simulink model "ADSBMonitor"  (R2022a)
settings: Solver=FixedStepDiscrete  StartTime=0.0  StopTime=10  RelTol=1e-3
PreLoadFcn:
  | radioSampleRate = 2.4e6;
  | adsbParam = helperAdsbConfig(radioSampleRate);
  | load dataAdsbBusObjects
  | LaunchMap = 0;
  | LogData = 0;
  | BaudRate=9600;
InitFcn:
  | load dataAdsbBusObjects
  | helperAdsbCheckModelParams;
libraries: simulink x2, ADSBExampleLib x2, commsource2 x1, sdrrlib x1
CloseFcn:
  | hFig = findall(0, 'Type', 'figure', 'Tag', 'ADS-B Aircraft Tracking');
  | if ishghandle(hFig)
  | close(hFig);
  | end
  | clear hFig
settings Model: Creator=The MathWorks, Inc.  LastModifiedBy=Michael
settings SolverCC: AlgebraicLoopSolver=TrustRegion
settings DataIOCC: LimitDataPoints=on  SaveFormat=Array  SaveOutput=off  SaveTime=off  ReturnWorkspaceOutputs=off
settings OptimizationCC: BooleanDataType=off  DefaultParameterBehavior=Inlined  LocalBlockOutputs=off  LifeSpan=inf
settings DebuggingCC: AlgebraicLoopMsg=error  SingleTaskRateTransMsg=error  UnconnectedInputMsg=warning  UnconnectedOutputMsg=warning  UnconnectedLineMsg=warning  AllowSymbolicDim=off  SFUnexpectedBacktrackingDiag=warning  SFNoUnconditionalDefaultTransitionDiag=warning  SFExecutionAtInitializationDiag=none  SFMachineParentedDataDiag=warning  ArithmeticOperatorsInVariantConditions=warning
settings ModelReferenceCC: PropagateSignalLabelsOutOfModel=off
settings SFSimCC: SimUseLocalCustomCode=off  CustomCodeUndefinedFunction=UseInterfaceOnly
settings RTWCC: RTWUseLocalCustomCode=off  DLArmComputeVersion=19.05
settings CodeAppCC: StateflowObjectComments=on
settings GRTTargetCC: TargetLangStandard=C89/C90 (ANSI)
settings ConfigComp: CovScope=ReferencedModels  CovMetricSettings=dw  CovSaveCumulativeToWorkspaceVar=on  CovSaveSingleToWorkspaceVar=on  CovExternalEMLEnable=off  CovSFcnEnable=off

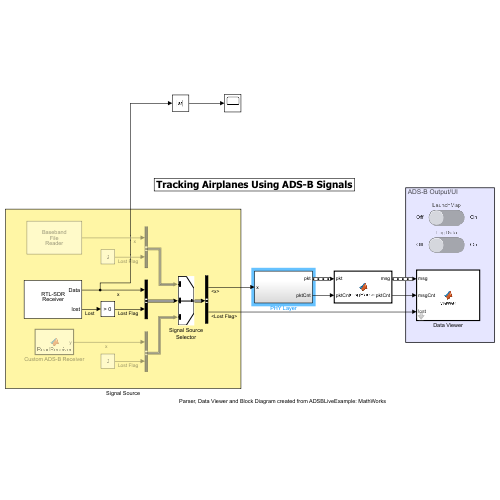
[thumbnail: Simulink's stored preview of the top-level diagram]
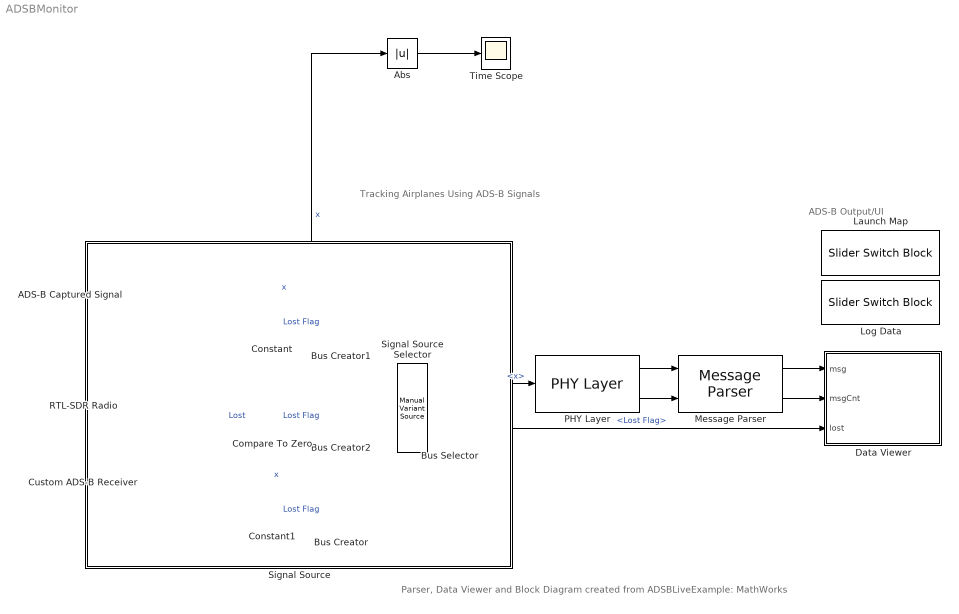
== system ADSBMonitor ==
  note: ADS-B Output/UI
  note: Tracking Airplanes Using ADS-B Signals
  note: Parser, Data Viewer and Block Diagram created from ADSBLiveExample: MathWorks
  ADS-B Captured Signal : commsource2/Baseband File Reader  Filename=adsb_capture_01.bb  InheritSampleTimeFromFile=on  SampleTime=1  SamplesPerFrame=adsbParam.SamplesPerFrame  CyclicRepetition=on  FileEndOutputPort=off  SimulateUsing=Code generation
      settings: SourceProductBaseCode=CM
  Abs : Abs  SaturateOnIntegerOverflow=off
  Bus Creator : BusCreator  Inputs=2
  Bus Creator1 : BusCreator  Inputs=2
  Bus Creator2 : BusCreator  Inputs=2
  Bus Selector : BusSelector  OutputSignals=x,Lost Flag
  Compare To Zero : simulink/Logic and Bit Operations/Compare To Zero  relop=>  OutDataTypeStr=boolean
  Constant : Constant  Value=0
  Constant1 : Constant  Value=0
  Custom ADS-B Receiver : MATLAB Function  TreatAsAtomicUnit=on
  Data Viewer : MATLAB Function  StopFcn=|  TreatAsAtomicUnit=on  mask(ADS-B viewer){logfilename=test.txt}
      | adsbGUI=findall(0,'type','figure','Tag','ADS-B Aircraft Tracking');
      | if ~isempty(adsbGUI)
      |   viewer=getappdata(adsbGUI,'ViewerHandle');
      |   stop(viewer);
      | end
      mask prompts: logfilename "Log data to file :"
  Launch Map : SliderSwitchBlock
      settings: Values={{'Off', 'On'}, [0 1]}
  Log Data : SliderSwitchBlock
      settings: Values={{'Off', 'On'}, [0 1]}
  Message Parser : ADSBExampleLib/Message Parser  SystemSampleTime=-1  VariantActivationTime=update diagram  Latency=0  AutoFrameSizeCalculation=off
  PHY Layer : ADSBExampleLib/PHY Layer  SystemSampleTime=-1  VariantActivationTime=update diagram  Latency=0  AutoFrameSizeCalculation=off
  RTL-SDR Radio : sdrrlib/RTL-SDR Receiver  IPAddress=0  CenterFrequencySource=Dialog  CenterFrequency=1090e6  GainSource=Dialog  Gain=60  ADCRate=adsbParam.FrontEndSampleRate  FrequencyCorrection=0  LostSamplesOutputPort=on  LatencyOutputPort=off  OutputDataType=single  FrameLength=adsbParam.SamplesPerFrame  EnableBurstMode=off  NumFramesInBurst=100  sobjType=sdrr.internal.SDRRTLReceiverSL  dataUDPPort=-1  ctrlUDPPort=-1  subDeviceList=nosubdev  sdrBlockType=SDRBlockTypeSLT.SDRRxBlock  requester=UNUSED_BY_SFCN  sdrExecutionMode=SDRExecutionModeSLT.ExecModeHW  BypassUserLogic=off  DecimatorSelect=DDC decimator  SourceSelect=RF data  SineAmplitude=16000  EnableInternalClock=off  BypassIQBalance=off  IFBandwidth=40e6  ADCRateSource=Dialog  IntermediateFrequency=0  DecimationFactorSource=Dialog  DecimationFactor=512  RFFrequencyIsTunable=logical(0)  SampleTime=(adsbParam.SamplesPerFrame)/(adsbParam.FrontEndSampleRate)  IFBandwidthSource=Dialog  SineFrequency=30000  BypassDCBlockingFilter=off  IntermediateFrequencySource=Dialog  IQBalanceCoefficients=64  SkipAllHardwareResetAndInitialization=off  EnableIQCalibrationTable=on  CacheIQCalibrationTable=off  EnableOffsetTuning=off  EnableRTLAGC=off  EnableTestMode=off  EnableTunerAGC=off  FrequencyCorrectionSource=Dialog  NumMLBuffers=128  NumUSBBuffers=16  RTLCrystalFrequency=28800000  TunerCrystalFrequency=28800000
      settings: SourceProductBaseCode=RTLSDR
  Signal Source : Subsystem
      mask Display: disp('')
  Signal Source Selector : simulink/Signal Routing/Manual Variant Source  NumChoices=3  LabelModeActiveChoice=V_2
  Time Scope : Scope
  wires:
  Message Parser/1 -> Data Viewer/1(msg)
  Message Parser/2 -> Data Viewer/2(msgCnt)
  PHY Layer/1 -> Message Parser/1
  PHY Layer/2 -> Message Parser/2
  Bus Selector/2 -> Data Viewer/3(lost)  "<Lost Flag>"
  Bus Selector/1 -> PHY Layer/1  "<x>"
  RTL-SDR Radio/1 -> Abs/1, Bus Creator2/1  "x"
  ADS-B Captured Signal/1 -> Bus Creator1/1  "x"
  Bus Creator2/1 -> Signal Source Selector/2
  Custom ADS-B Receiver/1(y) -> Bus Creator/1  "x"
  Signal Source Selector/1 -> Bus Selector/1
  Bus Creator/1 -> Signal Source Selector/3
  Bus Creator1/1 -> Signal Source Selector/1
  RTL-SDR Radio/2 -> Compare To Zero/1  "Lost"
  Compare To Zero/1 -> Bus Creator2/2  "Lost Flag"
  Constant/1 -> Bus Creator1/2  "Lost Flag"
  Constant1/1 -> Bus Creator/2  "Lost Flag"
  Abs/1 -> Time Scope/1

== system ADSBMonitor/Signal Source ==

== matlab function ADSBMonitor/Custom ADS-B Receiver ==
  data: y output
function y = ReadReceiver()
    %Ask User for port number 
    portnum=FindPort();
    %Create Serial Port Object
    feather=serialport(portnum,BaudRate);
    %Remove old data
    flush(feather);
    %Read Data and Output
    y = readline(src);
    %Save Output File to Binary File
    if LogData==0
        
    
end

%% Other Functions

%Ask User from menu to select desired serial port
function [feather_port]=FindPort()
   aval_ports=serialportlist('available');
   aval_ports=cellstr(aval_ports);
   [indx,~]=listdlg('ListString',aval_ports);
   feather_port=aval_ports{indx};               
end

== matlab function ADSBMonitor/Data Viewer ==
  data: msg input; msgCnt input; lost input; LaunchMap parameter; LogData parameter
function viewer(msg, msgCnt, lost, LaunchMap, LogData)
%#codegen

persistent resetGUI

if isempty(resetGUI)
  resetGUI = true;
end

block = 'ADSBMonitor/Data Viewer';

coder.extrinsic('helperAdsbViewerAdaptor');

coder.extrinsic('get_param','set_param');

Logfilename = get_param(block,'logfilename');

helperAdsbViewerAdaptor(msg, msgCnt, resetGUI, LaunchMap, LogData, Logfilename, lost);

resetGUI = false;
